simulink model "doc_pnseq2"  (R2014a)
settings: Solver=FixedStepDiscrete  SolverMode=SingleTasking  StartTime=0.0  StopTime=62  RelTol=1e-3
PreLoadFcn:
  | iniStates = [ 0 0 1 0 1 1];
undefined symbols (not defined in the file or in its folder): commblksprivate, Info
libraries: commseqgen2 x1
CloseFcn:
  | rtwprivate ssgencode ModelCloseRequest test1
settings Model: Creator=The MathWorks Inc.
settings DataIOCC: SignalLoggingSaveFormat=ModelDataLogs
settings OptimizationCC: ExpressionDepthLimit=2147483647  InitFltsAndDblsToZero=on  OptimizeModelRefInitCode=on  LifeSpan=1
settings DebuggingCC: SaveWithParameterizedLinksMsg=none  UnderspecifiedInitializationDetection=Classic  SignalResolutionControl=TryResolveAllWithWarning  MultiTaskDSMMsg=warning  MultiTaskCondExecSysMsg=none  FcnCallInpInsideContextMsg=UseLocalSettings  StateNameClashWarn=warning  StrictBusMsg=Warning
settings RTWCC: SystemTargetFile=ert.tlc  GenCodeOnly=on  TemplateMakefile=ert_default_tmf  Description=Real-Time Workshop Embedded Coder (no auto configuration)  ProcessScript=ert_make_rtw_hook  IncludeERTFirstTime=on
settings CodeAppCC: IgnoreCustomStorageClasses=off  CustomSymbolStrType=$N$R$M  InternalIdentifier=Classic
settings ERTTargetCC: TargetFcnLib=ansi_tfl_tmw.mat  ParMdlRefBuildCompliant=on  CompOptLevelCompliant=on  ConcurrentExecutionCompliant=on  ERTFirstTimeCompliant=on  ModelStepFunctionPrototypeControlCompliant=on  CPPClassGenCompliant=on  ERTCustomFileTemplate=example_file_process.tlc

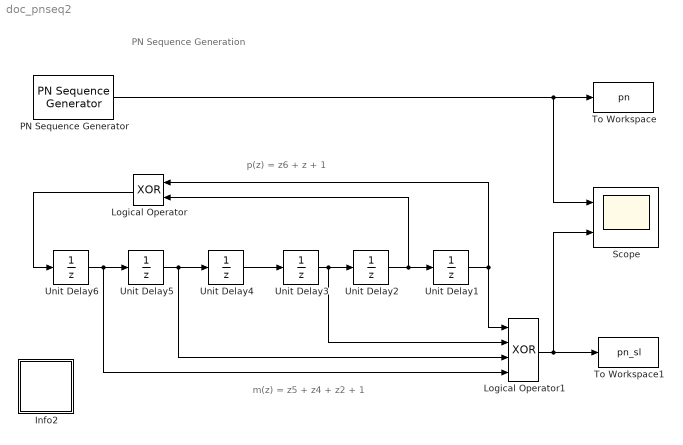
== system doc_pnseq2 ==
  note: PN Sequence Generation
  note: p(z) = z6 + z + 1
  note: m(z) = z5 + z4 + z2 + 1
  Info2 : Subsystem  AncestorBlock=commblksprivate/Info  mask(Info){}
      settings: OpenFcn=helpview([docroot '/toolbox/comm/comm.map'], 'doc_pnseq2')
      mask Display: disp('Info')
  Logical Operator : Logic  Operator=XOR  AllPortsSameDT=off  OutDataTypeStr=boolean
  Logical Operator1 : Logic  Operator=XOR  Inputs=4  AllPortsSameDT=off  OutDataTypeStr=boolean
  PN Sequence Generator : commseqgen2/PN Sequence Generator  poly=[1 0 0 0 0 1 1]  ini_sta=iniStates  outBitMaskSource=Dialog parameter  shift=[1 1 0 1 0 1]  outVarSiz=off  maxOutSizeMode=Dialog parameter  maxOutSize=[10 1]  Ts=1  frameBased=off  sampPerFrame=63  reset=off  bitPackedOutputs=off  outDataType=boolean  numPackedBits=8  bitPackDataSigned=off  bitPackedOutDType=double
  Scope : Scope  NumInputPorts=2
      settings: YMin=-5~-5  YMax=5~5
  To Workspace : ToWorkspace  VariableName=pn  SampleTime=-1
  To Workspace1 : ToWorkspace  VariableName=pn_sl  SampleTime=-1
  Unit Delay1 : UnitDelay  InitialCondition=iniStates(6)  SampleTime=-1
  Unit Delay2 : UnitDelay  InitialCondition=iniStates(5)  SampleTime=-1
  Unit Delay3 : UnitDelay  InitialCondition=iniStates(4)  SampleTime=-1
  Unit Delay4 : UnitDelay  InitialCondition=iniStates(3)  SampleTime=-1
  Unit Delay5 : UnitDelay  InitialCondition=iniStates(2)  SampleTime=-1
  Unit Delay6 : UnitDelay  InitialCondition=iniStates(1)  SampleTime=-1
  wires:
  PN Sequence Generator/1 -> Scope/1, To Workspace/1
  Logical Operator/1 -> Unit Delay6/1
  Unit Delay6/1 -> Unit Delay5/1, Logical Operator1/4
  Unit Delay5/1 -> Unit Delay4/1, Logical Operator1/3
  Unit Delay4/1 -> Unit Delay3/1
  Unit Delay3/1 -> Unit Delay2/1, Logical Operator1/2
  Unit Delay2/1 -> Unit Delay1/1, Logical Operator/2
  Unit Delay1/1 -> Logical Operator1/1, Logical Operator/1
  Logical Operator1/1 -> Scope/2, To Workspace1/1

== system doc_pnseq2/Info2 ==
